simulink model "spvonly"  (Simulink 7.5)
settings: Solver=ode45  StartTime=0.0  StopTime=0.1  RelTol=1e-3
undefined symbols (not defined in the file): Ts
libraries: powerlib x16
settings Model: Creator=sravan  LastModifiedBy=ACER LAP
settings DebuggingCC: StrictBusMsg=Warning

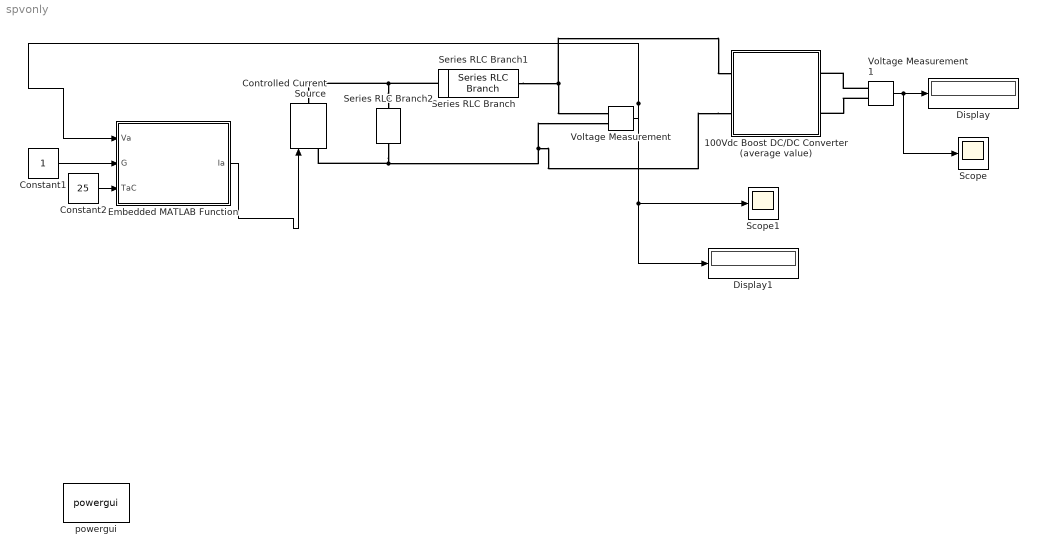
== system spvonly ==
  100Vdc Boost DC/DC Converter (average value) : Subsystem
  Constant1 : Constant  OutDataType=sfix(16)  OutScaling=2^0
  Constant2 : Constant  Value=25  OutDataType=sfix(16)  OutScaling=2^0
  Controlled Current Source : powerlib/Electrical Sources/Controlled Current Source  DialogController=POWERSYS.PowerSysDialog  SystemSampleTime=-1  Initialize=on  Source_Type=AC  Amplitude=0  Phase=0  Frequency=0  Measurements=None
  Display : Display
  Display1 : Display
  Embedded MATLAB Function : Stateflow chart  TreatAsAtomicUnit=on
  Scope : Scope
  Scope1 : Scope
  Series RLC Branch : powerlib/Elements/Series RLC Branch  DialogController=POWERSYS.PowerSysDialog  PhysicalDomain=powersysdomain  SubClassName=unknown  LeftPortType=p1  RightPortType=p1  LConnTagsString=__new0  RConnTagsString=__new0  BranchType=R  Resistance=0.005128  Inductance=1e-3  SetiL0=off  InitialCurrent=0  Capacitance=1e-6  Setx0=off  InitialVoltage=0  Measurements=None
  Series RLC Branch1 : powerlib/Elements/Series RLC Branch  DialogController=POWERSYS.PowerSysDialog  PhysicalDomain=powersysdomain  SubClassName=unknown  LeftPortType=p1  RightPortType=p1  LConnTagsString=__new0  RConnTagsString=__new0  BranchType=R  Resistance=0.005128  Inductance=1e-3  SetiL0=off  InitialCurrent=0  Capacitance=1e-6  Setx0=off  InitialVoltage=0  Measurements=None
  Series RLC Branch2 : powerlib/Elements/Series RLC Branch  DialogController=POWERSYS.PowerSysDialog  PhysicalDomain=powersysdomain  SubClassName=unknown  LeftPortType=p1  RightPortType=p1  LConnTagsString=__new0  RConnTagsString=__new0  BranchType=C  Resistance=0.00001  Inductance=1e-3  SetiL0=off  InitialCurrent=0  Capacitance=1e-6  Setx0=off  InitialVoltage=0  Measurements=None
  Voltage Measurement : powerlib/Measurements/Voltage Measurement  DialogController=POWERSYS.PowerSysDialog  SystemSampleTime=-1  PhasorSimulation=off  OutputType=Complex  PSBequivalent=0
  Voltage Measurement1 : powerlib/Measurements/Voltage Measurement  DialogController=POWERSYS.PowerSysDialog  SystemSampleTime=-1  PhasorSimulation=off  OutputType=Complex  PSBequivalent=0
  powergui : powerlib/powergui  Priority=1  SystemSampleTime=-1  SimulationMode=Continuous  SampleTime=50e-6  frequency=60  SPID=off  DisableSnubberDevices=off  DisableRonSwitches=off  DisableVfSwitches=off  SwTol=0  Interpol=off  frequencyindice=0  echomessages=off  HookPort=off  DisplayEquations=off  FunctionMessages=off  EnableUseOfTLC=off  x0status=blocks  RestoreLinks=warning  ResistiveCurrentMeasurement=off  Frange=[0:2:500]  Ylog=off  Xlog=on  ShowGrid=off  save=off  variable=ZData  ZoomFFT=on  StartTime=0.0  cycles=1  DisplayStyle=1  fundamental=60  FreqAxis=off  MaxFrequency=1000  frequencyindicesteady=1  RmsSteady=1  display=off  Ts=0  methode=off
  wires:
  Voltage Measurement/1 -> Embedded MATLAB Function/1(Va), Display1/1, Scope1/1
  Constant1/1 -> Embedded MATLAB Function/2(G)
  Constant2/1 -> Embedded MATLAB Function/3(TaC)
  Embedded MATLAB Function/1(Ia) -> Controlled Current Source/1
  Voltage Measurement1/1 -> Display/1, Scope/1
  connections:
  100Vdc Boost DC/DC Converter (average value)/LConn2 -- Controlled Current Source/LConn1 -- Series RLC Branch2/RConn1 -- Voltage Measurement/LConn2
  Series RLC Branch2/LConn1 -- Controlled Current Source/RConn1 -- Series RLC Branch/LConn1
  100Vdc Boost DC/DC Converter (average value)/LConn1 -- Voltage Measurement/LConn1 -- Series RLC Branch/RConn1
  Voltage Measurement1/LConn1 -- 100Vdc Boost DC/DC Converter (average value)/RConn1
  Voltage Measurement1/LConn2 -- 100Vdc Boost DC/DC Converter (average value)/RConn2

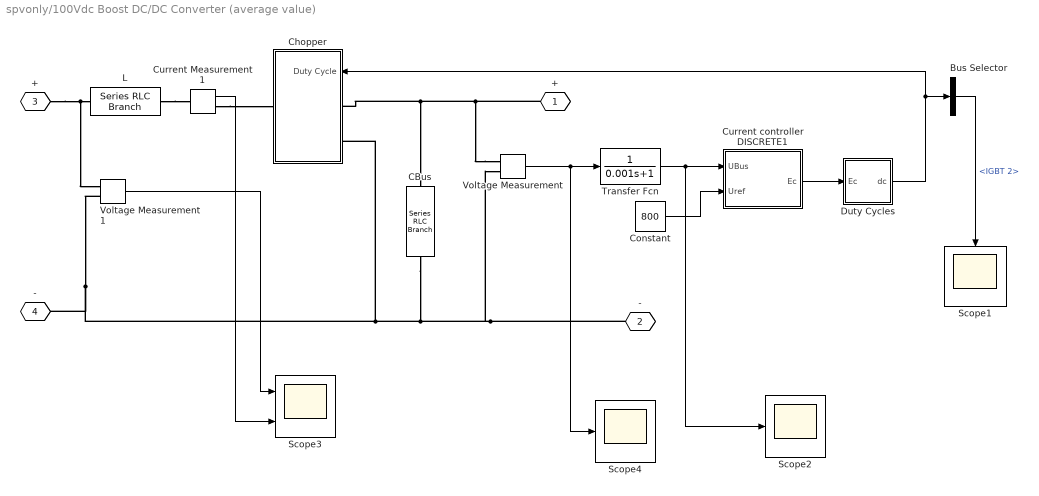
== system spvonly/100Vdc Boost DC/DC Converter (average value) ==
  Bus Selector : BusSelector  OutputSignals=IGBT 2
  CBus : powerlib/Elements/Series RLC Branch  DialogController=POWERSYS.PowerSysDialog  PhysicalDomain=powersysdomain  SubClassName=unknown  LeftPortType=p1  RightPortType=p1  LConnTagsString=__new0  RConnTagsString=__new0  BranchType=RC  Resistance=0.2  Inductance=1e-3  SetiL0=off  InitialCurrent=0  Capacitance=7500e-6  Setx0=on  InitialVoltage=100  Measurements=None
  Chopper : Subsystem  mask(SPSdrives Converter){SnubberResistance=10e3, SnubberCapacitance=inf, Ron=1e-3, ForwardVoltages=[1.3,1.3], IGBTParameters=[0,0], converterType=Inverter}
      mask prompts: SnubberResistance "Snubber resistance Rs (Ohms):"; SnubberCapacitance "Snubber capacitance Cs (F):"; Ron "Ron (Ohms):"; ForwardVoltages "Forward voltages [Device Vf(V), Diode Vd (V)]"; IGBTParameters "[Tf(s), Tt(s)]:"; converterType "Converter type:"
      mask help: This model implements an average-value buck converter."Duty Cycle" contains the duty cycle of the internal IGBT device.
      mask StyleString: edit,edit,edit,edit,edit,popup(Rectifier|Inverter)
      mask Display: plot(0,0,100,100,[39 39 23.8],[71 28 28],[44 56 49.6 56 52.8 56 61 61],[39.2 33.6 32.8 33.6 40.8 33.6 30 12.4],[44 44 44 61 61],[28 71 60 66.4 90],[75 67 83 75 67 83 75 75],[54 42 42 54 54 54 54 66],[61 75 75],[24 24 42],[75 75 61],[66,76,76])
  Constant : Constant  Value=800  OutDataType=sfix(16)  OutScaling=2^0
  Current Measurement1 : powerlib/Measurements/Current Measurement  DialogController=POWERSYS.PowerSysDialog  SystemSampleTime=-1  PhasorSimulation=off  OutputType=Complex  PSBequivalent=0
  Current controller DISCRETE1 : Subsystem  mask(PI controller){Kp=0.0005, Ki=0.15, Ts=Ts}
      mask prompts: Kp "Proportional gain (Kp)"; Ki "Integral gain (Ki)"; Ts "Sample time (s) :"
      mask help: Proportional-Integral Speed Controller
      mask Display: plot(0,0,100,100,[35,35,65],[70,30,30],[35,65],[45,60])
  Duty Cycles : Subsystem
  L : powerlib/Elements/Series RLC Branch  DialogController=POWERSYS.PowerSysDialog  PhysicalDomain=powersysdomain  SubClassName=unknown  LeftPortType=p1  RightPortType=p1  LConnTagsString=__new0  RConnTagsString=__new0  BranchType=L  Resistance=0.3  Inductance=500e-6  SetiL0=off  InitialCurrent=0  Capacitance=100e-6  Setx0=off  InitialVoltage=0  Measurements=None
  Scope1 : Scope
      settings: TimeRange=0.1  YMin=0.975  YMax=0.975  SaveName=ScopeData7
  Scope2 : Scope
      settings: TimeRange=0.5  YMin=699.88  YMax=700.04  SaveName=ScopeData20
  Scope3 : Scope  NumInputPorts=2
      settings: TimeRange=0.5  YMin=404.626~124.36  YMax=404.632~124.56  SaveName=ScopeData13
  Scope4 : Scope
      settings: TimeRange=0.5  YMin=695  YMax=725  SaveName=ScopeData6
  Transfer Fcn : TransferFcn  Denominator=[0.001 1]
  Voltage Measurement : powerlib/Measurements/Voltage Measurement  DialogController=POWERSYS.PowerSysDialog  SystemSampleTime=-1  PhasorSimulation=off  OutputType=Complex  PSBequivalent=0
  Voltage Measurement1 : powerlib/Measurements/Voltage Measurement  DialogController=POWERSYS.PowerSysDialog  SystemSampleTime=-1  PhasorSimulation=off  OutputType=Complex  PSBequivalent=0
  + : PMIOPort  Tag=PMCPort  Port=1  Side=Right
  - : PMIOPort  Tag=PMCPort  Port=2  Side=Right
  "+ " : PMIOPort  Tag=PMCPort  Port=3  Side=Left
  "- " : PMIOPort  Tag=PMCPort  Port=4  Side=Left
  wires:
  Constant/1 -> Current controller DISCRETE1/2(Uref)
  Voltage Measurement/1 -> Transfer Fcn/1, Scope4/1
  Transfer Fcn/1 -> Current controller DISCRETE1/1(UBus), Scope2/1
  Duty Cycles/1(dc) -> Chopper/1(Duty Cycle), Bus Selector/1
  Current controller DISCRETE1/1(Ec) -> Duty Cycles/1(Ec)
  Voltage Measurement1/1 -> Scope3/1
  Current Measurement1/1 -> Scope3/2
  Bus Selector/1 -> Scope1/1  "<IGBT 2>"
  connections:
  CBus/RConn1 -- -/RConn1 -- Voltage Measurement/LConn2 -- Voltage Measurement1/LConn2 -- "- "/RConn1 -- Chopper/LConn2
  Voltage Measurement/LConn1 -- +/RConn1 -- Chopper/LConn1 -- CBus/LConn1
  "+ "/RConn1 -- L/RConn1 -- Voltage Measurement1/LConn1
  L/LConn1 -- Current Measurement1/LConn1
  Current Measurement1/RConn1 -- Chopper/RConn1

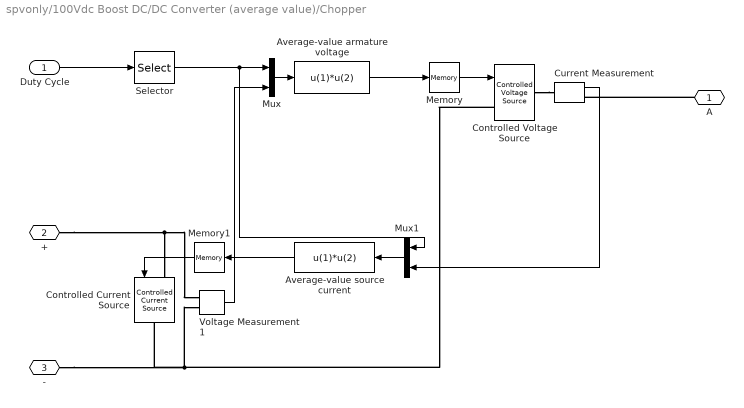
== system spvonly/100Vdc Boost DC/DC Converter (average value)/Chopper ==
  Duty Cycle : Inport  OutDataType=sfix(16)  OutScaling=2^0
  Average-value armature voltage : Fcn  Expr=u(1)*u(2)
  Average-value source current : Fcn  Expr=u(1)*u(2)
  Controlled Current Source : powerlib/Electrical Sources/Controlled Current Source  DialogController=POWERSYS.PowerSysDialog  SystemSampleTime=-1  Initialize=on  Source_Type=AC  Amplitude=0  Phase=0  Frequency=0  Measurements=None
  Controlled Voltage Source : powerlib/Electrical Sources/Controlled Voltage Source  DialogController=POWERSYS.PowerSysDialog  SystemSampleTime=-1  Initialize=on  Source_Type=AC  Amplitude=0  Phase=0  Frequency=0  Measurements=None
  Current Measurement : powerlib/Measurements/Current Measurement  Tag=PoWeRsYsTeMmEaSuReMeNt  DialogController=POWERSYS.PowerSysDialog  SystemSampleTime=-1  PhasorSimulation=off  OutputType=Magnitude  PSBequivalent=0
  Memory : Memory
  Memory1 : Memory
  Mux : Mux  Inputs=2
  Mux1 : Mux  Inputs=2
  Selector : Selector  InputPortWidth=2  IndexOptions=Index vector (dialog)  Indices=1  OutputSizes=1
  Voltage Measurement1 : powerlib/Measurements/Voltage Measurement  Tag=PoWeRsYsTeMmEaSuReMeNt  DialogController=POWERSYS.PowerSysDialog  SystemSampleTime=-1  PhasorSimulation=off  OutputType=Magnitude  PSBequivalent=0
  A : PMIOPort  Port=1  Side=Right
  + : PMIOPort  Port=2  Side=Left
  - : PMIOPort  Port=3  Side=Left
  wires:
  Selector/1 -> Mux1/1, Mux/1
  Memory1/1 -> Controlled Current Source/1
  Average-value source current/1 -> Memory1/1
  Current Measurement/1 -> Mux1/2
  Mux1/1 -> Average-value source current/1
  Duty Cycle/1 -> Selector/1
  Voltage Measurement1/1 -> Mux/2
  Mux/1 -> Average-value armature voltage/1
  Average-value armature voltage/1 -> Memory/1
  Memory/1 -> Controlled Voltage Source/1
  connections:
  A/RConn1 -- Current Measurement/RConn1
  Controlled Voltage Source/RConn1 -- Current Measurement/LConn1
  +/RConn1 -- Voltage Measurement1/LConn1 -- Controlled Current Source/LConn1
  Controlled Voltage Source/LConn1 -- -/RConn1 -- Controlled Current Source/RConn1 -- Voltage Measurement1/LConn2

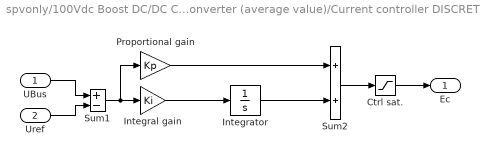
== system spvonly/100Vdc Boost DC/DC Converter (average value)/Current controller DISCRETE1 ==
  UBus : Inport  OutDataType=sfix(16)  OutScaling=2^0
  Uref : Inport  Port=2  OutDataType=sfix(16)  OutScaling=2^0
  Ctrl sat. : Saturate  UpperLimit=0.95  LowerLimit=-0.95
  Integral gain : Gain  Gain=Ki  ParameterDataType=sfix(16)  ParameterScaling=2^0  OutDataType=sfix(16)  OutScaling=2^0  SaturateOnIntegerOverflow=on  OutDataTypeStr=Inherit: Same as input  ParamDataTypeStr=Inherit: Same as input
  Integrator : Integrator
  Proportional gain : Gain  Gain=Kp  ParameterDataType=sfix(16)  ParameterScaling=2^0  OutDataType=sfix(16)  OutScaling=2^0  SaturateOnIntegerOverflow=on  OutDataTypeStr=Inherit: Same as input  ParamDataTypeStr=Inherit: Same as input
  Sum1 : Sum  Inputs=+-  OutDataType=sfix(16)  OutScaling=2^0  SaturateOnIntegerOverflow=on  InputSameDT=on  OutDataTypeStr=Inherit: Same as first input
  Sum2 : Sum  OutDataType=sfix(16)  OutScaling=2^0  SaturateOnIntegerOverflow=on  InputSameDT=on  OutDataTypeStr=Inherit: Same as first input
  Ec : Outport  OutDataType=sfix(16)  OutScaling=2^0  InitialOutput=0
  wires:
  Ctrl sat./1 -> Ec/1
  Sum2/1 -> Ctrl sat./1
  Integrator/1 -> Sum2/2
  Uref/1 -> Sum1/2
  UBus/1 -> Sum1/1
  Sum1/1 -> Proportional gain/1, Integral gain/1
  Integral gain/1 -> Integrator/1
  Proportional gain/1 -> Sum2/1

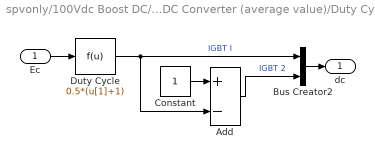
== system spvonly/100Vdc Boost DC/DC Converter (average value)/Duty Cycles ==
  Ec : Inport  OutDataType=sfix(16)  OutScaling=2^0
  Add : Sum  Inputs=+-  OutDataType=sfix(16)  OutScaling=2^-10
  Bus Creator2 : BusCreator  Inputs=2
  Constant : Constant  OutDataType=sfix(16)  OutScaling=2^0
  Duty Cycle : Fcn  Expr=0.5*(u[1]+1)  SampleTime=Ts
  dc : Outport  OutDataType=sfix(16)  OutScaling=2^0
  wires:
  Bus Creator2/1 -> dc/1
  Ec/1 -> Duty Cycle/1
  Constant/1 -> Add/1
  Add/1 -> Bus Creator2/2  "IGBT 2"
  Duty Cycle/1 -> Bus Creator2/1, Add/2  "IGBT I"

== matlab function Embedded MATLAB Function ==
  data: Va input double; Ia output double; G input double; TaC input double

function Ia = bp_sx150(Va,G,TaC)
%function bp_sx150s.m models the BP SX !%)S PV module
% calculates module current under given voltage, irradiance and temperature
% Ia= bp_sx150s(Va,G,T)
% 
%out: Ia= Module operating current (A), vector or scalar

k=1.381e-23;
q=1.602e-19;
n=1.62;
Eg=1.12;
Ns=72;
TrK=273+25;
Voc_TrK=43.5/Ns;
Isc_TrK=4.75;
a=0.65e-3;
TaK=273+TaC;
Isc=Isc_TrK*(1+(a*(TaK-TrK)));
Iph=G*Isc;
Vt_TrK=n*k*TrK/q;
b=Eg*q/(n*k);
Ir_TrK=Isc_TrK/(exp(Voc_TrK/Vt_TrK)-1);
Ir=Ir_TrK*(TaK/TrK)^(3/n)*exp(-b*(1/TaK-1/TrK));
dVdI_Voc=-1.0/Ns;
Xv=Ir_TrK/Vt_TrK*exp(Voc_TrK/Vt_TrK);
Rs=-dVdI_Voc-1/Xv;
Vt_Ta=n*k*TaK/q;
%Va1=linspace(0,Va,50);
%for i=1:length(Va1)
Vc=Va/Ns;
Ia=zeros(size(Vc));
for j=1:5
    Ia=Ia-(Iph-Ia-Ir .*(exp((Vc+Ia .*Rs) ./Vt_Ta)-1))./(-1-Ir*(Rs ./Vt_Ta) .*exp((Vc+Ia .*Rs) ./Vt_Ta));
end
